simulink model "Band_stop"  (R2018a)
settings: Solver=VariableStepAuto  StartTime=0.0  StopTime=0.01  RelTol=1e-3
libraries: dsparch4 x1
settings Model: Creator=AlexZ  LastModifiedBy=AlexZ

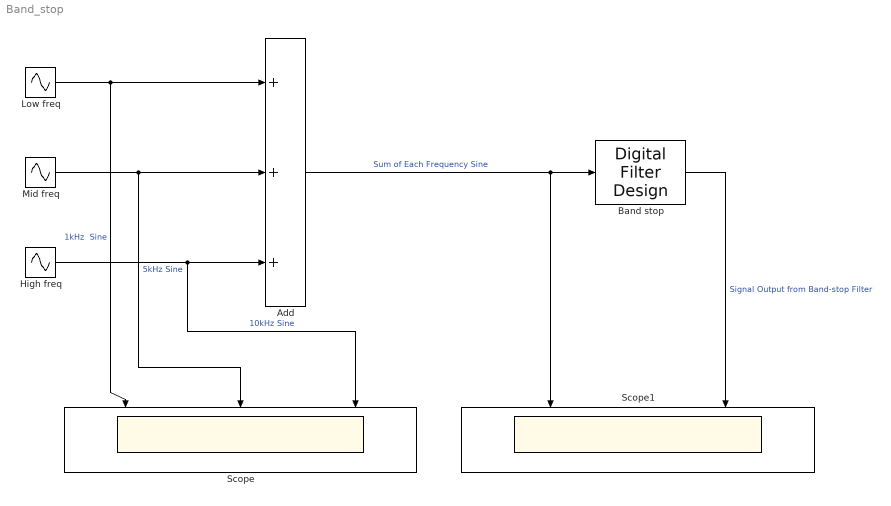
== system Band_stop ==
  Add : Sum  Inputs=+++
  "Band stop " : dsparch4/Digital Filter Design  mwdsp_browser_bugfix_var=off
  "High freq " : Sin  Frequency=2*pi*10000  Samples=1000  SampleTime=1e-6
  "Low freq " : Sin  Frequency=2*pi*1000  SampleTime=1e-6
  Mid freq : Sin  Frequency=2*pi*5000  SampleTime=1e-6  VectorParams1D=off
  Scope : Scope  NumInputPorts=3
  Scope1 : Scope  NumInputPorts=2
  wires:
  Add/1 -> "Band stop "/1, Scope1/1  "Sum of Each Frequency Sine"
  Mid freq/1 -> Scope/2, Add/2  "5kHz Sine"
  "High freq "/1 -> Scope/3, Add/3  "10kHz Sine"
  "Band stop "/1 -> Scope1/2  "Signal Output from Band-stop Filter"
  "Low freq "/1 -> Add/1, Scope/1  "1kHz  Sine"
